simulink model "Bridge_type_cycloconverter"  (R2023a)
settings: Solver=VariableStepAuto  StartTime=0.0  StopTime=10.0  RelTol=1e-3
libraries: spsThyristorLib x8, spsIdealSwitchLib x4, spsSeriesRLCBranchLib x3, spsVoltageMeasurementLib x2, spsACVoltageSourceLib x1, spsCurrentMeasurementLib x1, sps_lib x1
settings Model: Creator=Rudrajit  LastModifiedBy=Rudrajit

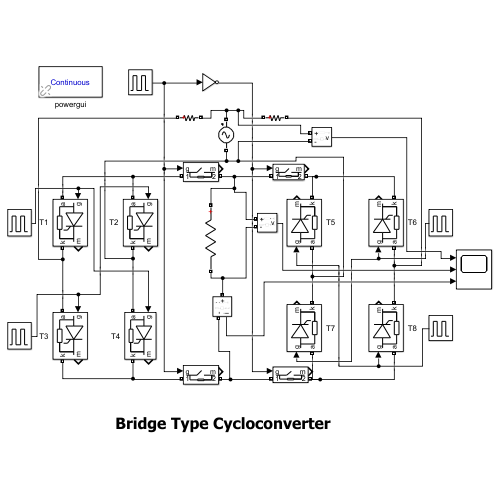
[thumbnail: Simulink's stored preview of the top-level diagram]
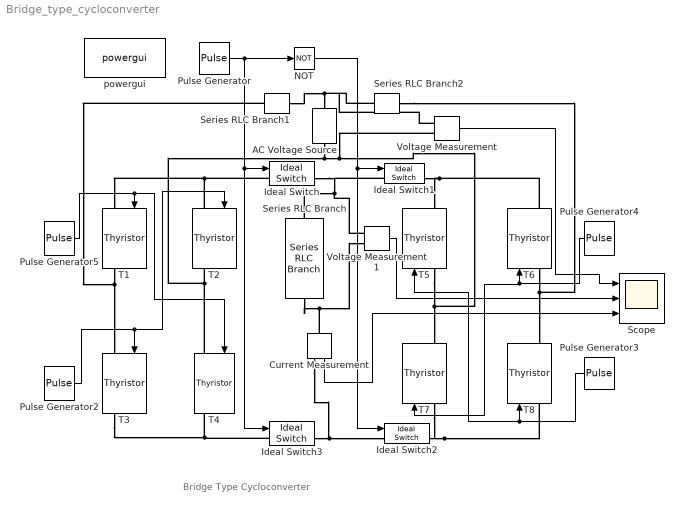
== system Bridge_type_cycloconverter ==
  note: Bridge Type Cycloconverter
  AC Voltage Source : spsACVoltageSourceLib/AC Voltage Source  Amplitude=100  Phase=0  Frequency=50  SampleTime=0  Measurements=None  BusType=swing  Pref=10e3  Qref=0  Qmin=-inf  Qmax=+inf
  Current Measurement : spsCurrentMeasurementLib/Current Measurement  PhasorSimulation=off  OutputType=Complex  PSBequivalent=0
  Ideal Switch{,1..3} (4 alike) : spsIdealSwitchLib/Ideal Switch  Ron=0.001  Lon=0  IC=0  Rs=1e5  Cs=inf  Measurements=on
  NOT : Logic  Operator=NOT  IconShape=distinctive  AllPortsSameDT=off  OutDataTypeStr=boolean
  Pulse Generator : DiscretePulseGenerator  PulseType=Time based  Period=0.06  PulseWidth=50
  Pulse Generator{2..5} (4 alike) : DiscretePulseGenerator  PulseType=Time based  Period=0.01  PulseWidth=5
  Scope : Scope  NumInputPorts=3
  Series RLC Branch : spsSeriesRLCBranchLib/Series RLC Branch  LConnTagsString=__new0  RConnTagsString=__new0  BranchType=R  Resistance=10  Inductance=1e-3  SetiL0=off  InitialCurrent=0  Capacitance=1e-6  Setx0=off  InitialVoltage=0  Measurements=None
  Series RLC Branch1 : spsSeriesRLCBranchLib/Series RLC Branch  LConnTagsString=__new0  RConnTagsString=__new0  BranchType=R  Resistance=10  Inductance=1e-3  SetiL0=off  InitialCurrent=0  Capacitance=1e-6  Setx0=off  InitialVoltage=0  Measurements=None
  Series RLC Branch2 : spsSeriesRLCBranchLib/Series RLC Branch  LConnTagsString=__new0  RConnTagsString=__new0  BranchType=R  Resistance=10  Inductance=1e-3  SetiL0=off  InitialCurrent=0  Capacitance=1e-6  Setx0=off  InitialVoltage=0  Measurements=None
  T{1..8} (8 alike) : spsThyristorLib/Thyristor  Ron=0.001  Lon=0  Vf=0.8  IC=0  Rs=500  Cs=250e-9  Measurements=on
  Voltage Measurement : spsVoltageMeasurementLib/Voltage Measurement  PhasorSimulation=off  OutputType=Complex  PSBequivalent=0
  Voltage Measurement1 : spsVoltageMeasurementLib/Voltage Measurement  PhasorSimulation=off  OutputType=Complex  PSBequivalent=0
  powergui : sps_lib/powergui  Priority=1  SimulationMode=Continuous  SampleTime=50e-6  frequency=60  Iterations=50  frequencyindice=50  Pbase=100e6  ErrMax=1e-4  UnitsV=kV  UnitsW=MW  buscounter=0  FunctionMessages=off  echomessages=off  EnableUseOfTLC=off  CurrentSourceSwitches=off  DisableSnubberDevices=off  DisableRonSwitches=off  DisableVfSwitches=off  DisplayEquations=off  AutomaticDiscreteSolvers=off  SolverType=Tustin/Backward Euler (TBE)  Interpol=off  ExternalGateDelay=off  methode=off  Ts=100  x0status=blocks  SPID=on  SwTol=0  HookPort=off  NonlinearTolerance=1e-4  nMaxIteration=100  ContinueOnMaxIteration=off  RestoreLinks=warning  ResistiveCurrentMeasurement=off  Frange=[0:2:500]  Ylog=off  Xlog=on  ShowGrid=off  save=off  variable=ZData  structure=0  ZoomFFT=off  StartTime=0.0  cycles=1  DisplayStyle=1  fundamental=60  FreqAxis=off  MaxFrequency=1000  frequencyindicesteady=1  RmsSteady=1  display=off
  wires:
  Voltage Measurement1/1 -> Scope/2
  Current Measurement/1 -> Scope/3
  Pulse Generator2/1 -> T2/1, T3/1
  Pulse Generator5/1 -> T4/1, T1/1
  Pulse Generator4/1 -> T7/1, T6/1
  Pulse Generator3/1 -> T8/1, T5/1
  Voltage Measurement/1 -> Scope/1
  Pulse Generator/1 -> NOT/1, Ideal Switch3/1, Ideal Switch/1
  NOT/1 -> Ideal Switch1/1, Ideal Switch2/1
  connections:
  T7/LConn1 -- T8/LConn1 -- Ideal Switch2/RConn1
  T2/LConn1 -- Ideal Switch/LConn1 -- T1/LConn1
  T1/RConn1 -- T3/LConn1 -- Series RLC Branch1/LConn1
  Series RLC Branch/RConn1 -- Voltage Measurement1/LConn2 -- Current Measurement/LConn1
  Voltage Measurement1/LConn1 -- Ideal Switch/RConn1 -- Ideal Switch1/LConn1 -- Series RLC Branch/LConn1
  T6/RConn1 -- T5/RConn1 -- Ideal Switch1/RConn1
  T3/RConn1 -- Ideal Switch3/LConn1 -- T4/RConn1
  Current Measurement/RConn1 -- Ideal Switch3/RConn1 -- Ideal Switch2/LConn1
  T6/LConn1 -- Series RLC Branch2/RConn1 -- T8/RConn1
  T4/LConn1 -- AC Voltage Source/LConn1 -- T7/RConn1 -- T5/LConn1 -- Voltage Measurement/LConn2 -- T2/RConn1
  Series RLC Branch1/RConn1 -- Series RLC Branch2/LConn1 -- Voltage Measurement/LConn1 -- AC Voltage Source/RConn1
